simulink model "PBA3_2"  (R2015a)
settings: Solver=ode45  StartTime=0.0  StopTime=10.0  RelTol=1e-3
values from neighbouring files (symbols this model uses):
  c = 0.08    [Bicycle_whipple.m]    (also in PBA3_2_script.m = 0.1; PBA3_4_script.m = 0.1)
  g = 9.81    [Bicycle_whipple.m]    (also in PBA1_script.m; PBA3_2_script.m; PBA3_4_script.m; cruise_control.m)
  l = 1    [PBA3_2_script.m]    (also in PBA3_4_script.m)
  M = [Jxxt -Flx-gamma*Jxzt;-Flx-gamma*Jxzt Fll+2*gamma*Flz+gamma^2*Jzzt]    [Bicycle_whipple.m]    (also in PBA3_2_script.m = 10; PBA3_4_script.m = 10)
  m = 1200    [PBA1_script.m]    (also in PBA3_2_script.m = 80; PBA3_4_script.m = 80; cruise_control.m = 1000)
  rho = 0.01    [PBA3_2_script.m]    (also in PBA3_4_script.m; helicopter_eom.m = sym('rho(t)'))
settings Model: Creator=Callum  LastModifiedBy=Callum
settings DataIOCC: LimitDataPoints=off
settings HardwareCC: TargetLongLongMode=on  TargetIntDivRoundTo=Zero  TargetEndianess=LittleEndian  TargetHWDeviceType=MATLAB Host  ProdEqTarget=off
settings RTWCC: SystemTargetFile=rsim.tlc  TemplateMakefile=rsim_default_tmf  Description=Rapid Simulation Target
settings RSimTargetCC: ERTMultiwordTypeDef=System defined  ERTMultiwordLength=256

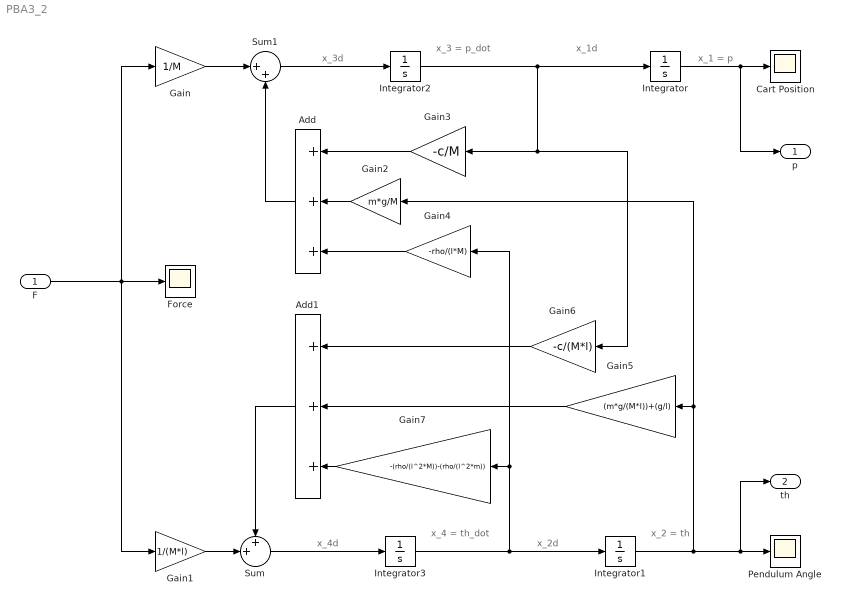
== system PBA3_2 ==
  note: x_2 = th
  note: x_2d
  note: x_1 = p
  note: x_1d
  note: x_3 = p_dot
  note: x_3d
  note: x_4 = th_dot
  note: x_4d
  F : Inport
  Add : Sum  Inputs=+++
  Add1 : Sum  Inputs=+++
  Cart Position : Scope
  Force : Scope
      settings: SaveName=ScopeData2
  Gain : Gain  Gain=1/M
  Gain1 : Gain  Gain=1/(M*l)
  Gain2 : Gain  Gain=m*g/M
  Gain3 : Gain  Gain=-c/M
  Gain4 : Gain  Gain=-rho/(l*M)
  Gain5 : Gain  Gain=(m*g/(M*l))+(g/l)
  Gain6 : Gain  Gain=-c/(M*l)
  Gain7 : Gain  Gain=-(rho/(l^2*M))-(rho/(l^2*m))
  Integrator{,1..3} (4 alike) : Integrator
  Pendulum Angle : Scope
  Sum : Sum  Inputs=++|
  Sum1 : Sum  Inputs=|++
  p : Outport
  th : Outport  Port=2
  wires:
  Integrator/1 -> p/1, Cart Position/1
  Integrator3/1 -> Gain4/1, Gain7/1, Integrator1/1
  Integrator1/1 -> Gain2/1, Gain5/1, th/1, Pendulum Angle/1
  F/1 -> Force/1, Gain/1, Gain1/1
  Sum1/1 -> Integrator2/1
  Integrator2/1 -> Gain3/1, Gain6/1, Integrator/1
  Sum/1 -> Integrator3/1
  Gain/1 -> Sum1/1
  Add/1 -> Sum1/2
  Gain3/1 -> Add/1
  Gain2/1 -> Add/2
  Gain4/1 -> Add/3
  Gain1/1 -> Sum/2
  Gain5/1 -> Add1/2
  Gain6/1 -> Add1/1
  Gain7/1 -> Add1/3
  Add1/1 -> Sum/1
